simulink model "Woodward_v9_milestone"  (Simulink 7.8)
settings: Solver=ode5  StartTime=0.0  StopTime=inf  FixedStep=Ts  MaxStep=1e-3  RelTol=1e-3
PostLoadFcn:
  | Ts=50e-6;
InitFcn:
  | Ts=50e-6;
undefined symbols (not defined in the file): another_event_name, dfilt, DiscIntNeverNeededParam, fdesignblkfcn, gcbh, Gen_900kW_external_control, HIL_GenSet, Left, my_event_name, ph, type, V
libraries: simulink x66, powerlib x65, rtio_opalrt_common x21, powerlib_extras x20, dspsigops x10, simulink_extras x6, cables_lib x5, discretizing x4, rteventslib x4, dsparch4 x4, rtlab x3, ssn_lib x2
(part 1 of 5)
settings Model: ARTEMISmethode_block_infos=$$__separator__$$  Creator=CH24070  LastModifiedBy=ma25949  BufferReuse=off
settings SolverCC: ZeroCrossAlgorithm=Adaptive
settings DataIOCC: ExternalInput=getinputstruct(op_snapshot1)  InitialState=getstatestruct(op_snapshot1)  LimitDataPoints=off  MaxDataPoints=90060  SignalLoggingSaveFormat=Dataset  SaveOutput=off  SignalLogging=off  DSMLogging=off  SaveTime=off  OutputSaveName=result
settings OptimizationCC: BlockReduction=off  OptimizeBlockIOStorage=off  BufferReuse=off  ExpressionFolding=off  LocalBlockOutputs=off
settings DebuggingCC: MaxConsecutiveZCsMsg=warning  IgnoredZcDiagnostic=none  SolverPrmCheckMsg=none  MultiTaskRateTransMsg=warning  FrameProcessingCompatibilityMsg=error  ModelReferenceExtraNoncontSigs=warning
settings ModelReferenceCC: UpdateModelReferenceTargets=IfOutOfDate
settings SFSimCC: SFSimEcho=off
settings CodeAppCC: CustomSymbolStrType=$N$R$M_T
settings GRTTargetCC: TargetFunctionLibrary=C89/C90 (ANSI)
settings CustomProperty: DataType=string  Value=0

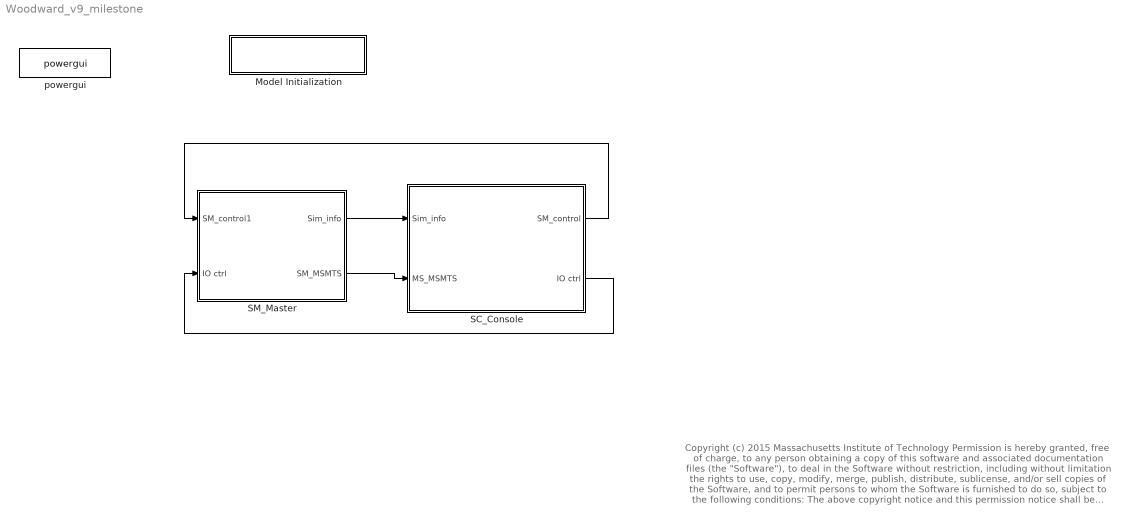
== system Woodward_v9_milestone ==
  note: Copyright (c) 2015 Massachusetts Institute of Technology
      | Permission is hereby granted, free of charge, to any person obtaining a copy of this software and associated documentation files (the "Software"), to deal in the Software without restriction, including without limitation the rights to use, copy, modify, merge, publish, distribute, sublicense, and/or sell copies of the Software, and to permit persons to whom the Software is furnished to do so, subject to the following conditions:
      |
      | The above copyright notice and this permission notice shall be included in all copies or substantial portions of the Software.
      |
      | THE SOFTWARE IS PROVIDED "AS IS", WITHOUT WARRANTY OF ANY KIND, EXPRESS OR IMPLIED, INCLUDING BUT NOT LIMITED TO THE WARRANTIES OF MERCHANTABILITY, FITNESS FOR A PARTICULAR PURPOSE AND NONINFRINGEMENT. IN NO EVENT SHALL THE AUTHORS OR COPYRIGHT HOLDERS BE LIABLE FOR ANY CLAIM,
      | DAMAGES OR OTHER LIABILITY, WHETHER IN AN ACTION OF CONTRACT, TORT OR OTHERWISE, ARISING FROM, OUT OF OR IN CONNECTION WITH THE SOFTWARE OR THE USE OR OTHER DEALINGS IN THE SOFTWARE.
  Model Initialization : Subsystem  AncestorBlock=artemis/Tools /Misc/Model Initialization  mask(Model Functions){InitFcnX=Ts=50e-6;, prel=off, posl=on, inif=on, strf=off}
      mask prompts: InitFcnX "Initialisation"; prel "Preload Function"; posl "PostLoad Function"; inif "InitFcn"; strf "StartFcn"
      mask init:
      | currentBlock = gcb;
      | root = bdroot(currentBlock);
      | 
      | if ~strcmp(get_param(root,'BlockDiagramType'),'library')
      |     if prel==1
      |         set_param(root, 'PreLoadFcn', InitFcnX);
      |     else
      |         set_param(root, 'PreLoadFcn', '');
      |     end
      |     if inif==1
      |         set_param(root, 'InitFcn', InitFcnX);
      |     else
      |         set_param(root, 'InitFcn', '');
      |     end
      |     if strf==1
      |         set_param(root, 'StartFcn', InitFcnX);
      |     else
      |         set_param(root, 'StartFcn', '');
      |     end
      |     if posl==1
      |         set_param(root, 'PostLoadFcn', InitFcnX);
      |     else
      |         set_param(root, 'PostLoadFcn', '');
      |     end
      | end
      | 
      | pos = get_param(currentBlock, 'Position');
      | width = pos(3) - pos(1); height = pos(4) - pos(2);
      | txt = [ upper(root) '\n' '- InitFcn. . . . . '  get_param(root, 'InitFcn') ];
      settings: CopyFcn=set_param(gcb,'LinkStatus','inactive')
      mask Display: text(5, height*0.5, txt, 'horizontalAlignment', 'left', 'verticalAlignment', 'middle') ;
  SC_Console : Subsystem
  SM_Master : Subsystem
  powergui : powerlib/powergui  Priority=2  SimulationMode=Discrete  SolverType=Tustin  SampleTime=Ts  frequency=60  SPID=off  DisableSnubberDevices=off  DisableRonSwitches=off  DisableVfSwitches=off  SwTol=0  Interpol=off  DisplayEquations=off  FunctionMessages=off  frequencyindice=0  Pbase=100e6  ErrMax=1e-4  Iterations=50  UnitsV=kV  UnitsW=MW  echomessages=off  HookPort=off  EnableUseOfTLC=off  x0status=blocks  RestoreLinks=warning  ResistiveCurrentMeasurement=off  Frange=logspace(0,3,50)  Ylog=off  Xlog=off  ShowGrid=off  save=off  variable=ZData  structure=0  ZoomFFT=on  StartTime=0.0  cycles=2  DisplayStyle=off  fundamental=60  FreqAxis=off  MaxFrequency=1000  frequencyindicesteady=1  RmsSteady=1  display=off  Ts=0  methode=off
  wires:
  SM_Master/1(Sim_info) -> SC_Console/1(Sim_info)
  SM_Master/2(SM_MSMTS) -> SC_Console/2(MS_MSMTS)
  SC_Console/1(SM_control) -> SM_Master/1(SM_control1)
  SC_Console/2(IO ctrl) -> SM_Master/2(IO ctrl)

== system Woodward_v9_milestone/Model Initialization ==

== system Woodward_v9_milestone/SC_Console ==
  note: Tcomputation
      | Ttotal
      | Idle
      | Overruns
  note: The 'Overruns' value should remain at 0.
      | The 'Ttotal' value should be equal to the
      | model Fixed-Step size.
  Sim_info : Inport
  MS_MSMTS : Inport  Port=2
  Bus Creator : BusCreator  Inputs=2
  Bus Selector : BusSelector  OutputSignals=Grid_PRM,Mains1_PRM,GEN_1MVA_PRM,Mains2_PRM,GEN_4MVA_PRM,Gen1_meas,Gen2_meas,Digital In,Load1,Load2,Load3
  Bus Selector{1..8} (8 alike) : BusSelector  OutputSignals=Grid_Status,sel_787.Grid_Vabc,sel_787.Iabc,sel_787.Grid_P,sel_787.Grid_Q
  Demux5 : Demux  Outputs=[1 8 4]
  Gen1_1MVA : Subsystem  AncestorBlock=HIL_GenSet/Gen_900kW_external_control
  Gen2_4MVA : Subsystem  AncestorBlock=HIL_GenSet/Gen_900kW_external_control
  OpComm : rtlab/OpComm  nbport=2  groupe_acq=1  subsys_rate=0  st=0  Synchronization=on  Interpolation=on  Threshold=1.0  Missed_Data=off  Sim_Time=off  Samples=off  dynSigOut=off  from_console=0  warning_done=off  writeOpCommFile=off  Offset=off
  Scope Gen1 : Scope  NumInputPorts=5
      settings: TimeRange=60  YMin=0~-600~-2000~-1000000~-1000000  YMax=1~600~2000~1000000~1000000
  Scope Gen2 : Scope  NumInputPorts=5
      settings: TimeRange=60  YMin=0~-20000~-20000~-1000000~-1000000  YMax=1~20000~20000~4000000~4000000  SaveName=ScopeData8
  Scope Grid : Scope  NumInputPorts=5
      settings: TimeRange=60  YMin=0~-20000~-20000~-1000000~-1000000  YMax=1~20000~20000~4000000~4000000  SaveName=ScopeData7
  Scope Load1 : Scope  NumInputPorts=5
      settings: TimeRange=60  YMin=0~-600~-2000~-1000000~-1000000  YMax=1~600~2000~1000000~1000000  SaveName=ScopeData6
  Scope Load2 : Scope  NumInputPorts=5
      settings: TimeRange=60  YMin=0~-600~-2000~-1000000~-1000000  YMax=1~600~2000~1000000~1000000  SaveName=ScopeData11
  Scope Load3 : Scope  NumInputPorts=5
      settings: TimeRange=60  YMin=0~-600~-2000~-1000000~-1000000  YMax=1~600~2000~1000000~1000000  SaveName=ScopeData10
  Scope Mains1 : Scope  NumInputPorts=5
      settings: TimeRange=60  YMin=0~-20000~-20000~-1000000~-1000000  YMax=1~20000~20000~4000000~4000000  SaveName=ScopeData5
  Scope Mains2 : Scope  NumInputPorts=5
      settings: TimeRange=60  YMin=0~-20000~-20000~-1000000~-1000000  YMax=1~20000~20000~4000000~4000000  SaveName=ScopeData9
  Status Codes : Display
      settings: Decimation=100
  TimingValues : Display
      settings: Decimation=100
  Woodward : Subsystem
  SM_control : Outport
  IO ctrl : Outport  Port=2
  wires:
  Sim_info/1 -> OpComm/1
  MS_MSMTS/1 -> OpComm/2
  Gen1_1MVA/1(S) -> Bus Creator/1  "Gen1_1MVA"
  Bus Creator/1 -> SM_control/1
  OpComm/2 -> Bus Selector/1
  Demux5/3 -> TimingValues/1
  OpComm/1 -> Demux5/1
  Demux5/1 -> Status Codes/1
  Woodward/1(Out1) -> IO ctrl/1
  Bus Selector1/1 -> Scope Grid/1  "<Grid_Status>"
  Bus Selector1/2 -> Scope Grid/2  "<Grid_Vabc>"
  Bus Selector1/3 -> Scope Grid/3  "<Iabc>"
  Bus Selector1/4 -> Scope Grid/4  "<Grid_P>"
  Bus Selector1/5 -> Scope Grid/5  "<Grid_Q>"
  Bus Selector2/1 -> Scope Mains1/1  "<Grid_Status>"
  Bus Selector2/2 -> Scope Mains1/2  "<Grid_Vabc>"
  Bus Selector2/3 -> Scope Mains1/3  "<Iabc>"
  Bus Selector2/4 -> Scope Mains1/4  "<Grid_P>"
  Bus Selector2/5 -> Scope Mains1/5  "<Grid_Q>"
  Bus Selector/1 -> Bus Selector1/1  "<Grid_PRM>"
  Bus Selector/2 -> Bus Selector2/1  "<Mains1_PRM>"
  Bus Selector3/1 -> Scope Load1/1  "<Grid_Status>"
  Bus Selector3/2 -> Scope Load1/2  "<Grid_Vabc>"
  Bus Selector3/3 -> Scope Load1/3  "<Iabc>"
  Bus Selector3/4 -> Scope Load1/4  "<Grid_P>"
  Bus Selector3/5 -> Scope Load1/5  "<Grid_Q>"
  Bus Selector/9 -> Bus Selector3/1  "<Load1>"
  Bus Selector4/1 -> Scope Gen1/1  "<Grid_Status>"
  Bus Selector4/2 -> Scope Gen1/2  "<Grid_Vabc>"
  Bus Selector4/3 -> Scope Gen1/3  "<Iabc>"
  Bus Selector4/4 -> Scope Gen1/4  "<Grid_P>"
  Bus Selector4/5 -> Scope Gen1/5  "<Grid_Q>"
  Bus Selector/3 -> Bus Selector4/1  "<GEN_1MVA_PRM>"
  Bus Selector5/1 -> Scope Gen2/1  "<Grid_Status>"
  Bus Selector5/2 -> Scope Gen2/2  "<Grid_Vabc>"
  Bus Selector5/3 -> Scope Gen2/3  "<Iabc>"
  Bus Selector5/4 -> Scope Gen2/4  "<Grid_P>"
  Bus Selector5/5 -> Scope Gen2/5  "<Grid_Q>"
  Bus Selector/5 -> Bus Selector5/1  "<GEN_4MVA_PRM>"
  Bus Selector/6 -> Woodward/1(Gen1_Primary)  "<Gen1_meas>"
  Bus Selector/8 -> Woodward/3(DIn_Ch00_31)  "<Digital In>"
  Bus Selector/7 -> Woodward/2(Gen2_Primary)  "<Gen2_meas>"
  Gen2_4MVA/1(S) -> Bus Creator/2  "Gen2_4MVA"
  Bus Selector6/1 -> Scope Mains2/1  "<Grid_Status>"
  Bus Selector6/2 -> Scope Mains2/2  "<Grid_Vabc>"
  Bus Selector6/3 -> Scope Mains2/3  "<Iabc>"
  Bus Selector6/4 -> Scope Mains2/4  "<Grid_P>"
  Bus Selector/4 -> Bus Selector6/1  "<Mains2_PRM>"
  Bus Selector6/5 -> Scope Mains2/5  "<Grid_Q>"
  Bus Selector7/1 -> Scope Load3/1  "<Grid_Status>"
  Bus Selector7/2 -> Scope Load3/2  "<Grid_Vabc>"
  Bus Selector7/3 -> Scope Load3/3  "<Iabc>"
  Bus Selector7/4 -> Scope Load3/4  "<Grid_P>"
  Bus Selector7/5 -> Scope Load3/5  "<Grid_Q>"
  Bus Selector8/1 -> Scope Load2/1  "<Grid_Status>"
  Bus Selector8/2 -> Scope Load2/2  "<Grid_Vabc>"
  Bus Selector8/3 -> Scope Load2/3  "<Iabc>"
  Bus Selector8/4 -> Scope Load2/4  "<Grid_P>"
  Bus Selector8/5 -> Scope Load2/5  "<Grid_Q>"
  Bus Selector/11 -> Bus Selector7/1  "<Load3>"
  Bus Selector/10 -> Bus Selector8/1  "<Load2>"

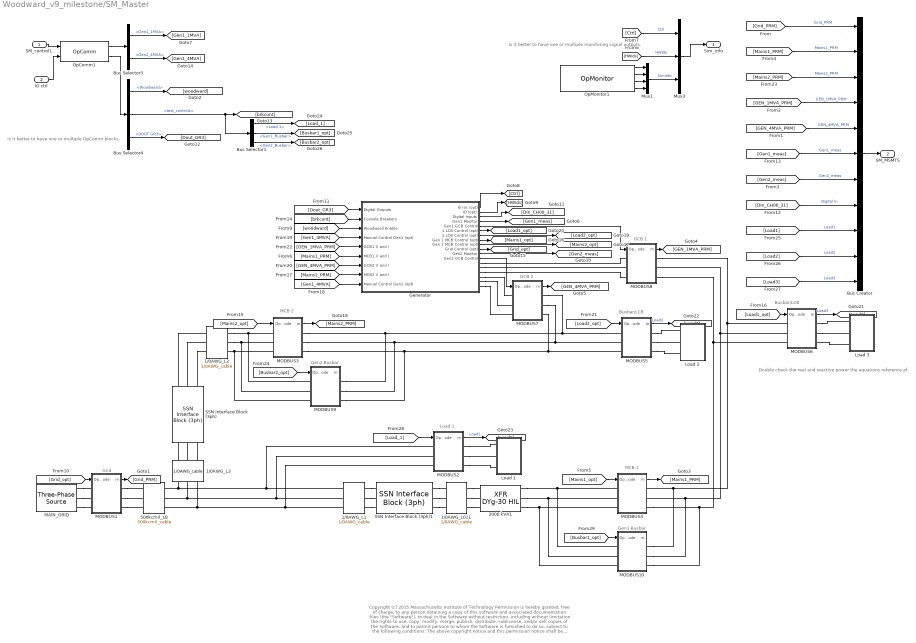
== system Woodward_v9_milestone/SM_Master ==
  note: Double check the real and reactive power
      | the equations reference pf.
  note: Is it better to have one
      | or multiple OpComm blocks.
  note: Is it better to have one or multiple
      | monitoring signal outputs.
  note: GCB 1
  note: Busbar/LCB
  note: MCB 1
  note: Grid
  note: MCB 2
  note: GCB 2
  note: Load 1
  note: Busbar/LCB
  note: Gen2 Busbar
  note: Gen1 Busbar
  note: Copyright (c) 2015 Massachusetts Institute of Technology
      | Permission is hereby granted, free of charge, to any person obtaining a copy of this software and associated documentation files (the "Software"), to deal in the Software without restriction, including without limitation the rights to use, copy, modify, merge, publish, distribute, sublicense, and/or sell copies of the Software, and to permit persons to whom the Software is furnished to do so, subject to the following conditions:
      |
      | The above copyright notice and this permission notice shall be included in all copies or substantial portions of the Software.
      |
      | THE SOFTWARE IS PROVIDED "AS IS", WITHOUT WARRANTY OF ANY KIND, EXPRESS OR IMPLIED, INCLUDING BUT NOT LIMITED TO THE WARRANTIES OF MERCHANTABILITY, FITNESS FOR A PARTICULAR PURPOSE AND NONINFRINGEMENT. IN NO EVENT SHALL THE AUTHORS OR COPYRIGHT HOLDERS BE LIABLE FOR ANY CLAIM,
      | DAMAGES OR OTHER LIABILITY, WHETHER IN AN ACTION OF CONTRACT, TORT OR OTHERWISE, ARISING FROM, OUT OF OR IN CONNECTION WITH THE SOFTWARE OR THE USE OR OTHER DEALINGS IN THE SOFTWARE.
  SM_control1 : Inport
  IO ctrl : Inport  Port=2
  1/0AWG_L011 : cables_lib/1//0AWG_cable  length=1000  par_sets=1
  1/0AWG_L1 : cables_lib/1//0AWG_cable  length=1  par_sets=1
  1/0AWG_L2 : cables_lib/1//0AWG_cable  length=1  par_sets=1
  1/0AWG_L3 : cables_lib/1//0AWG_cable  length=1  par_sets=1
  2000 kVA1 : transformer_lib/XFR DYg-30 HIL  Rating=2000  Vp=13800  Vs=480  Z=5.75  XR=5.7
  500kcmil_L8 : cables_lib/500kcmil_cable  length=1  par_sets=1
  Bus Creator : BusCreator  Inputs=11
  Bus Selector1 : BusSelector  OutputSignals=Load 1,Gen1_Busbar,Gen2_Busbar
  Bus Selector3 : BusSelector  OutputSignals=Gen1_1MVA,Gen2_4MVA
  Bus Selector4 : BusSelector  OutputSignals=Woodward,test_controls,DOUT GR3
  Generator : Subsystem
  Load 1 : Subsystem  mask{v=13800, kVA=1000, pf=0.90}
      mask prompts: v "VRMSLL"
  Load 2 : Subsystem  mask{v=13800, kVA=2000, pf=0.90}
      mask prompts: v "VRMSLL"
  Load 3 : Subsystem  mask{v=480, kVA=500, pf=0.90}
      mask prompts: v "VRMSLL"
  MAIN_GRID : powerlib/Electrical Sources/Three-Phase Source  Voltage=13800  PhaseAngle=0  Frequency=60  InternalConnection=Yg  SpecifyImpedance=on  Resistance=0.8929  Inductance=16.58e-3  ShortCircuitLevel=375e6  BaseVoltage=13800  XRratio=7.9  BusType=swing  Pref=0  Qref=0  Qmin=-inf  Qmax=inf
  MODBUS1 : Subsystem  mask(Protection and Metering){IOC=15E3, TOC=1800, Ts=Ts, VRMSLL=13800, I_nom=200}
      mask prompts: IOC "IOC setting [A]"; TOC "TOC setting [A]"; Ts "Sampling Time [Sec]"; VRMSLL "Nominal Voltage [VRMSLL]"; I_nom "Continous Current [A]"
      mask help:
      | This block simulates the behavior of selected relay functions as well as metering equipment.
      | The block is intended to communicate with a microgrid controller providing it measurements, and switching controls.
      mask Help:
      | This block simulates the behavior of selected relay functions as well as metering equipment (60 Hz - only).
      | The block is intended to communicate with a microgrid controller providing it measurements, and switching controls.
      | 
      | The input parameters are:
      | 0) Ts:  Sampling time [Seconds]
      | 1) State: 0 for relay logic mode, 1 to close the controlled breaker/switch,
      | and 2 to open the controlled breaker/switch
      | 2) TOC: Time-inverse overcurrent setting [Amperes]
      | 3) IOC: Instantaneous overcurrent setting [Amperes]
      | 
      | Metered parameters are:
      | 0) Status (0-closed, 1-open)
      | 1) Instantaneous voltage (abc)
      | 2) Instantaneous current (abc)
  MODBUS10 : Subsystem  mask(Protection and Metering){IOC=15E3, TOC=1800, Ts=Ts, VRMSLL=480, I_nom=2000}
      mask prompts: IOC "IOC setting [A]"; TOC "TOC setting [A]"; Ts "Sampling Time [Sec]"; VRMSLL "Nominal Voltage [VRMSLL]"; I_nom "Continous Current [A]"
      mask help:
      | This block simulates the behavior of selected relay functions as well as metering equipment.
      | The block is intended to communicate with a microgrid controller providing it measurements, and switching controls.
      mask Help:
      | This block simulates the behavior of selected relay functions as well as metering equipment (60 Hz - only).
      | The block is intended to communicate with a microgrid controller providing it measurements, and switching controls.
      | 
      | The input parameters are:
      | 0) Ts:  Sampling time [Seconds]
      | 1) State: 0 for relay logic mode, 1 to close the controlled breaker/switch,
      | and 2 to open the controlled breaker/switch
      | 2) TOC: Time-inverse overcurrent setting [Amperes]
      | 3) IOC: Instantaneous overcurrent setting [Amperes]
      | 
      | Metered parameters are:
      | 0) Status (0-closed, 1-open)
      | 1) Instantaneous voltage (abc)
      | 2) Instantaneous current (abc)
  MODBUS2 : Subsystem  mask(Protection and Metering){IOC=15E3, TOC=1800, Ts=Ts, VRMSLL=13800, I_nom=200}
      mask prompts: IOC "IOC setting [A]"; TOC "TOC setting [A]"; Ts "Sampling Time [Sec]"; VRMSLL "Nominal Voltage [VRMSLL]"; I_nom "Continous Current [A]"
      mask help:
      | This block simulates the behavior of selected relay functions as well as metering equipment.
      | The block is intended to communicate with a microgrid controller providing it measurements, and switching controls.
      mask Help:
      | This block simulates the behavior of selected relay functions as well as metering equipment (60 Hz - only).
      | The block is intended to communicate with a microgrid controller providing it measurements, and switching controls.
      | 
      | 
      | The input parameters are:
      | 0) Ts:  Sampling time [Seconds]
      | 1) State: 0 for relay logic mode, 1 to close the controlled breaker/switch,
      | and 2 to open the controlled breaker/switch
      | 2) TOC: Time-inverse overcurrent setting [Amperes]
      | 3) IOC: Instantaneous overcurrent setting [Amperes]
      | 
      | Metered parameters are:
      | 0) Status (0-closed, 1-open)
      | 1) Instantaneous voltage (abc)
      | 2) Instantaneous current (abc)
  MODBUS3 : Subsystem  mask(Protection and Metering){IOC=15E3, TOC=1800, Ts=Ts, VRMSLL=13800, I_nom=200}
      mask prompts: IOC "IOC setting [A]"; TOC "TOC setting [A]"; Ts "Sampling Time [Sec]"; VRMSLL "Nominal Voltage [VRMSLL]"; I_nom "Continous Current [A]"
      mask help:
      | This block simulates the behavior of selected relay functions as well as metering equipment.
      | The block is intended to communicate with a microgrid controller providing it measurements, and switching controls.
      mask Help:
      | This block simulates the behavior of selected relay functions as well as metering equipment (60 Hz - only).
      | The block is intended to communicate with a microgrid controller providing it measurements, and switching controls.
      | 
      | The input parameters are:
      | 0) Ts:  Sampling time [Seconds]
      | 1) State: 0 for relay logic mode, 1 to close the controlled breaker/switch,
      | and 2 to open the controlled breaker/switch
      | 2) TOC: Time-inverse overcurrent setting [Amperes]
      | 3) IOC: Instantaneous overcurrent setting [Amperes]
      | 
      | Metered parameters are:
      | 0) Status (0-closed, 1-open)
      | 1) Instantaneous voltage (abc)
      | 2) Instantaneous current (abc)
  MODBUS4 : Subsystem  mask(Protection and Metering){IOC=15E3, TOC=1800, Ts=Ts, VRMSLL=480, I_nom=2000}
      mask prompts: IOC "IOC setting [A]"; TOC "TOC setting [A]"; Ts "Sampling Time [Sec]"; VRMSLL "Nominal Voltage [VRMSLL]"; I_nom "Continous Current [A]"
      mask help:
      | This block simulates the behavior of selected relay functions as well as metering equipment.
      | The block is intended to communicate with a microgrid controller providing it measurements, and switching controls.
      mask Help:
      | This block simulates the behavior of selected relay functions as well as metering equipment (60 Hz - only).
      | The block is intended to communicate with a microgrid controller providing it measurements, and switching controls.
      | 
      | The input parameters are:
      | 0) Ts:  Sampling time [Seconds]
      | 1) State: 0 for relay logic mode, 1 to close the controlled breaker/switch,
      | and 2 to open the controlled breaker/switch
      | 2) TOC: Time-inverse overcurrent setting [Amperes]
      | 3) IOC: Instantaneous overcurrent setting [Amperes]
      | 
      | Metered parameters are:
      | 0) Status (0-closed, 1-open)
      | 1) Instantaneous voltage (abc)
      | 2) Instantaneous current (abc)
  MODBUS5 : Subsystem  mask(Protection and Metering){IOC=15E3, TOC=1800, Ts=Ts, VRMSLL=13800, I_nom=200}
      mask prompts: IOC "IOC setting [A]"; TOC "TOC setting [A]"; Ts "Sampling Time [Sec]"; VRMSLL "Nominal Voltage [VRMSLL]"; I_nom "Continous Current [A]"
      mask help:
      | This block simulates the behavior of selected relay functions as well as metering equipment.
      | The block is intended to communicate with a microgrid controller providing it measurements, and switching controls.
      mask Help:
      | This block simulates the behavior of selected relay functions as well as metering equipment (60 Hz - only).
      | The block is intended to communicate with a microgrid controller providing it measurements, and switching controls.
      | 
      | The input parameters are:
      | 0) Ts:  Sampling time [Seconds]
      | 1) State: 0 for relay logic mode, 1 to close the controlled breaker/switch,
      | and 2 to open the controlled breaker/switch
      | 2) TOC: Time-inverse overcurrent setting [Amperes]
      | 3) IOC: Instantaneous overcurrent setting [Amperes]
      | 
      | Metered parameters are:
      | 0) Status (0-closed, 1-open)
      | 1) Instantaneous voltage (abc)
      | 2) Instantaneous current (abc)
  MODBUS6 : Subsystem  mask(Protection and Metering){IOC=15E3, TOC=1800, Ts=Ts, VRMSLL=13800, I_nom=200}
      mask prompts: IOC "IOC setting [A]"; TOC "TOC setting [A]"; Ts "Sampling Time [Sec]"; VRMSLL "Nominal Voltage [VRMSLL]"; I_nom "Continous Current [A]"
      mask help:
      | This block simulates the behavior of selected relay functions as well as metering equipment.
      | The block is intended to communicate with a microgrid controller providing it measurements, and switching controls.
      mask Help:
      | This block simulates the behavior of selected relay functions as well as metering equipment (60 Hz - only).
      | The block is intended to communicate with a microgrid controller providing it measurements, and switching controls.
      | 
      | The input parameters are:
      | 0) Ts:  Sampling time [Seconds]
      | 1) State: 0 for relay logic mode, 1 to close the controlled breaker/switch,
      | and 2 to open the controlled breaker/switch
      | 2) TOC: Time-inverse overcurrent setting [Amperes]
      | 3) IOC: Instantaneous overcurrent setting [Amperes]
      | 
      | Metered parameters are:
      | 0) Status (0-closed, 1-open)
      | 1) Instantaneous voltage (abc)
      | 2) Instantaneous current (abc)
  MODBUS7 : Subsystem  mask(Protection and Metering){IOC=15E3, TOC=1800, Ts=Ts, VRMSLL=13800, I_nom=200}
      mask prompts: IOC "IOC setting [A]"; TOC "TOC setting [A]"; Ts "Sampling Time [Sec]"; VRMSLL "Nominal Voltage [VRMSLL]"; I_nom "Continous Current [A]"
      mask help:
      | This block simulates the behavior of selected relay functions as well as metering equipment.
      | The block is intended to communicate with a microgrid controller providing it measurements, and switching controls.
      mask Help:
      | This block simulates the behavior of selected relay functions as well as metering equipment (60 Hz - only).
      | The block is intended to communicate with a microgrid controller providing it measurements, and switching controls.
      | 
      | The input parameters are:
      | 0) Ts:  Sampling time [Seconds]
      | 1) State: 0 for relay logic mode, 1 to close the controlled breaker/switch,
      | and 2 to open the controlled breaker/switch
      | 2) TOC: Time-inverse overcurrent setting [Amperes]
      | 3) IOC: Instantaneous overcurrent setting [Amperes]
      | 
      | Metered parameters are:
      | 0) Status (0-closed, 1-open)
      | 1) Instantaneous voltage (abc)
      | 2) Instantaneous current (abc)
  MODBUS8 : Subsystem  mask(Protection and Metering){IOC=15E3, TOC=1800, Ts=Ts, VRMSLL=480, I_nom=2000}
      mask prompts: IOC "IOC setting [A]"; TOC "TOC setting [A]"; Ts "Sampling Time [Sec]"; VRMSLL "Nominal Voltage [VRMSLL]"; I_nom "Continous Current [A]"
      mask help:
      | This block simulates the behavior of selected relay functions as well as metering equipment.
      | The block is intended to communicate with a microgrid controller providing it measurements, and switching controls.
      mask Help:
      | This block simulates the behavior of selected relay functions as well as metering equipment (60 Hz - only).
      | The block is intended to communicate with a microgrid controller providing it measurements, and switching controls.
      | 
      | The input parameters are:
      | 0) Ts:  Sampling time [Seconds]
      | 1) State: 0 for relay logic mode, 1 to close the controlled breaker/switch,
      | and 2 to open the controlled breaker/switch
      | 2) TOC: Time-inverse overcurrent setting [Amperes]
      | 3) IOC: Instantaneous overcurrent setting [Amperes]
      | 
      | Metered parameters are:
      | 0) Status (0-closed, 1-open)
      | 1) Instantaneous voltage (abc)
      | 2) Instantaneous current (abc)
  MODBUS9 : Subsystem  mask(Protection and Metering){IOC=15E3, TOC=1800, Ts=Ts, VRMSLL=13800, I_nom=200}
      mask prompts: IOC "IOC setting [A]"; TOC "TOC setting [A]"; Ts "Sampling Time [Sec]"; VRMSLL "Nominal Voltage [VRMSLL]"; I_nom "Continous Current [A]"
      mask help:
      | This block simulates the behavior of selected relay functions as well as metering equipment.
      | The block is intended to communicate with a microgrid controller providing it measurements, and switching controls.
      mask Help:
      | This block simulates the behavior of selected relay functions as well as metering equipment (60 Hz - only).
      | The block is intended to communicate with a microgrid controller providing it measurements, and switching controls.
      | 
      | 
      | The input parameters are:
      | 0) Ts:  Sampling time [Seconds]
      | 1) State: 0 for relay logic mode, 1 to close the controlled breaker/switch,
      | and 2 to open the controlled breaker/switch
      | 2) TOC: Time-inverse overcurrent setting [Amperes]
      | 3) IOC: Instantaneous overcurrent setting [Amperes]
      | 
      | Metered parameters are:
      | 0) Status (0-closed, 1-open)
      | 1) Instantaneous voltage (abc)
      | 2) Instantaneous current (abc)
  Mux1 : Mux
  Mux3 : Mux  Inputs=[1 8 4]
  OpComm1 : rtlab/OpComm  nbport=2  groupe_acq=1  subsys_rate=0  st=0  Synchronization=on  Interpolation=on  Threshold=1.0  Missed_Data=off  Sim_Time=off  Samples=off  dynSigOut=off  from_console=1  warning_done=off  writeOpCommFile=off  Offset=off
  OpMonitor1 : rtlab/Monitoring/OpMonitor  compute_time=on  real_step=on  idle_time=on  nb_overruns=on  user_time=off  user_name=my_event_name,another_event_name
  SSN Interface Block (3ph) : ssn_lib/SSN Interface Block (3ph)  nb_phase=3  nb_port=2  p1_type=V-type(Left)  p2_type=V-type (Right)  p3_type=V-type(Left)  p4_type=V-type(Left)  p5_type=V-type(Left)  p6_type=V-type(Left)  p7_type=V-type(Left)  p8_type=V-type(Left)  p9_type=V-type(Left)  p10_type=V-type(Left)  p11_type=V-type(Left)  p12_type=V-type(Left)  p13_type=V-type(Left)  p14_type=V-type(Left)  p15_type=V-type(Left)  p16_type=V-type(Left)  I_port_shunt_resistance=1e9
  SSN Interface Block (3ph)1 : ssn_lib/SSN Interface Block (3ph)  nb_phase=3  nb_port=2  p1_type=V-type(Left)  p2_type=V-type (Right)  p3_type=V-type(Left)  p4_type=V-type(Left)  p5_type=V-type(Left)  p6_type=V-type(Left)  p7_type=V-type(Left)  p8_type=V-type(Left)  p9_type=V-type(Left)  p10_type=V-type(Left)  p11_type=V-type(Left)  p12_type=V-type(Left)  p13_type=V-type(Left)  p14_type=V-type(Left)  p15_type=V-type(Left)  p16_type=V-type(Left)  I_port_shunt_resistance=1e9
  Sim_info : Outport
  SM_MSMTS : Outport  Port=2
  wires:
  [Grid_PRM] -> Bus Creator/1  "Grid_PRM"
  [GEN_1MVA_PRM] -> Bus Creator/4  "GEN_1MVA_PRM"
  [Mains1_PRM] -> Bus Creator/2  "Mains1_PRM"
  Bus Creator/1 -> SM_MSMTS/1
  SM_control1/1 -> OpComm1/1
  OpComm1/1 -> Bus Selector3/1
  Bus Selector3/1 -> [Gen1_1MVA]  "<Gen1_1MVA>"
  OpComm1/2 -> Bus Selector4/1
  Bus Selector4/1 -> [woodward]  "<Woodward>"
  IO ctrl/1 -> OpComm1/2
  Bus Selector4/3 -> [Dout_GR3]  "<DOUT GR3>"
  OpMonitor1/1 -> Mux1/1
  OpMonitor1/2 -> Mux1/2
  OpMonitor1/3 -> Mux1/3
  OpMonitor1/4 -> Mux1/4
  Mux1/1 -> Mux3/3  "SimInfo"
  [Ctrl] -> Mux3/1  "Ctrl"
  [HWIds] -> Mux3/2  "HWIds"
  Mux3/1 -> Sim_info/1
  Bus Selector4/2 -> [brkcont], Bus Selector1/1  "<test_controls>"
  MODBUS1/1(m) -> [Grid_PRM]
  MODBUS8/1(m) -> [GEN_1MVA_PRM]
  [Dout_GR3] -> Generator/1(Digital Outputs)
  [brkcont] -> Generator/2(Console Breakers)
  Generator/4(Gen1 Monitor) -> [Gen1_meas]
  Generator/1(Error (opt)) -> [Ctrl]
  Generator/2(ID (opt)) -> [HWIds]
  Generator/3(Digital Inputs) -> [DIn_CH00_31]
  [Gen1_4MVA] -> Generator/4(Manual Control Gen1 (opt))
  [woodward] -> Generator/3(Woodward Enable)
  Generator/5(Gen1 GCB Control) -> MODBUS8/1(Op_Mode)
  Generator/12(Gen2 GCB Control) -> MODBUS7/1(Op_Mode)
  [GEN_4MVA_PRM] -> Bus Creator/5  "GEN_4MVA_PRM"
  Generator/11(Gen2 Monitor) -> [Gen2_meas]
  [Gen1_meas] -> Bus Creator/6  "Gen1_meas"
  [Gen2_meas] -> Bus Creator/7  "Gen2_meas"
  [DIn_CH00_31] -> Bus Creator/8  "Digital In"
  Bus Selector3/2 -> [Gen1_4MVA]  "<Gen2_4MVA>"
  [Gen1_4MVA] -> Generator/9(Manual Control Gen2 (opt))
  Generator/10(Grid Control (opt)) -> [Grid_opt]
  [Grid_opt] -> MODBUS1/1(Op_Mode)
  Generator/8(Gen 1 MCB Control (opt)) -> [Mains1_opt]
  Generator/9(Gen 2 MCB Control (opt)) -> [Mains2_opt]
  [Mains2_opt] -> MODBUS3/1(Op_Mode)
  MODBUS3/1(m) -> [Mains2_PRM]
  [Mains2_PRM] -> Generator/8(MCB2 V and I)
  [Mains1_PRM] -> Generator/6(MCB1 V and I)
  Generator/7(2 LCB Control (opt)) -> [Load2_opt]
  Generator/6(1 LCB Control (opt)) -> [Load1_opt]
  MODBUS7/1(m) -> [GEN_4MVA_PRM]
  [GEN_4MVA_PRM] -> Generator/7(GCB2 V and I)
  [GEN_1MVA_PRM] -> Generator/5(GCB1 V and I)
  [Mains2_PRM] -> Bus Creator/3  "Mains2_PRM"
  MODBUS4/1(m) -> [Mains1_PRM]
  [Mains1_opt] -> MODBUS4/1(Op_Mode)
  [Load2_opt] -> MODBUS5/1(Op_Mode)
  [Load1_opt] -> MODBUS6/1(Op_Mode)
  MODBUS2/1(m) -> [Load1]  "Load1"
  MODBUS5/1(m) -> [Load2]  "Load2"
  MODBUS6/1(m) -> [Load3]  "Load3"
  [Load1] -> Bus Creator/9  "Load1"
  [Load2] -> Bus Creator/10  "Load2"
  [Load3] -> Bus Creator/11  "Load3"
  Bus Selector1/1 -> [Load_1]  "<Load 1>"
  Bus Selector1/2 -> [Busbar1_opt]  "<Gen1_Busbar>"
  Bus Selector1/3 -> [Busbar2_opt]  "<Gen2_Busbar>"
  [Busbar2_opt] -> MODBUS9/1(Op_Mode)
  [Load_1] -> MODBUS2/1(Op_Mode)
  [Busbar1_opt] -> MODBUS10/1(Op_Mode)
  connections:
  1/0AWG_L011/RConn1 -- 2000 kVA1/LConn1
  1/0AWG_L011/RConn2 -- 2000 kVA1/LConn2
  1/0AWG_L011/RConn3 -- 2000 kVA1/LConn3
  1/0AWG_L1/LConn1 -- MODBUS2/LConn1 -- 500kcmil_L8/RConn1 -- 1/0AWG_L3/LConn1
  1/0AWG_L1/LConn2 -- MODBUS2/LConn2 -- 500kcmil_L8/RConn2 -- 1/0AWG_L3/LConn2
  1/0AWG_L1/LConn3 -- MODBUS2/LConn3 -- 500kcmil_L8/RConn3 -- 1/0AWG_L3/LConn3
  MODBUS4/RConn3 -- MODBUS6/LConn3 -- MODBUS8/RConn3 -- MODBUS10/RConn3
  MODBUS1/RConn3 -- 500kcmil_L8/LConn3
  MODBUS1/RConn2 -- 500kcmil_L8/LConn2
  MODBUS1/RConn1 -- 500kcmil_L8/LConn1
  MAIN_GRID/RConn3 -- MODBUS1/LConn3
  MAIN_GRID/RConn2 -- MODBUS1/LConn2
  MAIN_GRID/RConn1 -- MODBUS1/LConn1
  Generator/RConn3 -- MODBUS8/LConn3
  Generator/RConn2 -- MODBUS8/LConn2
  Generator/RConn1 -- MODBUS8/LConn1
  Generator/RConn6 -- MODBUS7/LConn3
  Generator/RConn5 -- MODBUS7/LConn2
  Generator/RConn4 -- MODBUS7/LConn1
  MODBUS2/RConn3 -- Load 1/LConn3
  MODBUS2/RConn2 -- Load 1/LConn2
  MODBUS2/RConn1 -- Load 1/LConn1
  MODBUS6/LConn2 -- MODBUS8/RConn2 -- MODBUS4/RConn2 -- MODBUS10/RConn2
  MODBUS6/LConn1 -- MODBUS8/RConn1 -- MODBUS4/RConn1 -- MODBUS10/RConn1
  MODBUS3/RConn3 -- MODBUS5/LConn3 -- MODBUS7/RConn3 -- MODBUS9/RConn3
  MODBUS3/RConn2 -- MODBUS5/LConn2 -- MODBUS7/RConn2 -- MODBUS9/RConn2
  MODBUS3/RConn1 -- MODBUS5/LConn1 -- MODBUS7/RConn1 -- MODBUS9/RConn1
  2000 kVA1/RConn3 -- MODBUS4/LConn3 -- MODBUS10/LConn3
  2000 kVA1/RConn2 -- MODBUS4/LConn2 -- MODBUS10/LConn2
  2000 kVA1/RConn1 -- MODBUS4/LConn1 -- MODBUS10/LConn1
  MODBUS5/RConn3 -- Load 2/LConn3
  MODBUS5/RConn2 -- Load 2/LConn2
  MODBUS5/RConn1 -- Load 2/LConn1
  MODBUS6/RConn3 -- Load 3/LConn3
  MODBUS6/RConn2 -- Load 3/LConn2
  MODBUS6/RConn1 -- Load 3/LConn1
  SSN Interface Block (3ph)1/RConn1 -- 1/0AWG_L011/LConn1
  SSN Interface Block (3ph)1/RConn2 -- 1/0AWG_L011/LConn2
  SSN Interface Block (3ph)1/RConn3 -- 1/0AWG_L011/LConn3
  1/0AWG_L1/RConn3 -- SSN Interface Block (3ph)1/LConn3
  1/0AWG_L1/RConn2 -- SSN Interface Block (3ph)1/LConn2
  1/0AWG_L1/RConn1 -- SSN Interface Block (3ph)1/LConn1
  MODBUS9/LConn3 -- MODBUS3/LConn3 -- 1/0AWG_L2/RConn3
  MODBUS9/LConn2 -- MODBUS3/LConn2 -- 1/0AWG_L2/RConn2
  MODBUS9/LConn1 -- MODBUS3/LConn1 -- 1/0AWG_L2/RConn1
  SSN Interface Block (3ph)/RConn3 -- 1/0AWG_L2/LConn3
  SSN Interface Block (3ph)/RConn2 -- 1/0AWG_L2/LConn2
  SSN Interface Block (3ph)/RConn1 -- 1/0AWG_L2/LConn1
  1/0AWG_L3/RConn3 -- SSN Interface Block (3ph)/LConn3
  1/0AWG_L3/RConn2 -- SSN Interface Block (3ph)/LConn2
  1/0AWG_L3/RConn1 -- SSN Interface Block (3ph)/LConn1

== system Woodward_v9_milestone/SC_Console/Gen1_1MVA ==
  1 - PQ 2 - PV 3 - VF : Constant  Value=3
  Bus Creator : BusCreator  Inputs=6
  DONOTCHANGE : Constant
  Enable = 1 Disable = 0 : Constant  Value=0
  F : simulink/Math Operations/Slider Gain  low=0.97  gain=1  high=1.03
  P : simulink/Math Operations/Slider Gain  low=0  gain=0.8  high=1.1
  Q : simulink/Math Operations/Slider Gain  low=0.01  gain=0.2  high=0.4
  V : simulink/Math Operations/Slider Gain  low=0.9  gain=1  high=1.1
  S : Outport
  wires:
  DONOTCHANGE/1 -> P/1, Q/1, V/1, F/1
  Bus Creator/1 -> S/1
  P/1 -> Bus Creator/1  "P"
  Q/1 -> Bus Creator/2  "Q"
  V/1 -> Bus Creator/3  "V"
  F/1 -> Bus Creator/4  "F"
  1 - PQ 2 - PV 3 - VF/1 -> Bus Creator/5  "Mode"
  Enable = 1 Disable = 0/1 -> Bus Creator/6  "Enable"

== system Woodward_v9_milestone/SC_Console/Gen2_4MVA ==
  1 - PQ 2 - PV 3 - VF : Constant  Value=3
  Bus Creator : BusCreator  Inputs=6
  DONOTCHANGE : Constant
  Enable = 1 Disable = 0 : Constant  Value=0
  F : simulink/Math Operations/Slider Gain  low=0.97  gain=1  high=1.03
  P : simulink/Math Operations/Slider Gain  low=0  gain=0.8  high=1.1
  Q : simulink/Math Operations/Slider Gain  low=0.01  gain=0.2  high=0.4
  V : simulink/Math Operations/Slider Gain  low=0.9  gain=1  high=1.1
  S : Outport
  wires:
  DONOTCHANGE/1 -> P/1, Q/1, V/1, F/1
  Bus Creator/1 -> S/1
  P/1 -> Bus Creator/1  "P"
  Q/1 -> Bus Creator/2  "Q"
  V/1 -> Bus Creator/3  "V"
  F/1 -> Bus Creator/4  "F"
  1 - PQ 2 - PV 3 - VF/1 -> Bus Creator/5  "Mode"
  Enable = 1 Disable = 0/1 -> Bus Creator/6  "Enable"

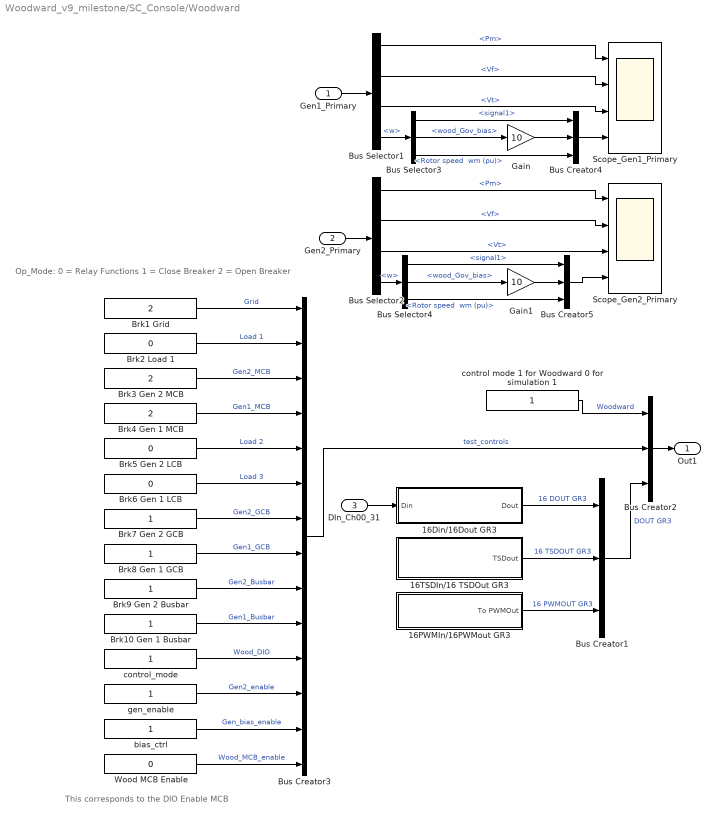
== system Woodward_v9_milestone/SC_Console/Woodward ==
  note: Op_Mode:
      | 0 = Relay Functions
      | 1 = Close Breaker
      | 2 = Open Breaker
  note: This corresponds to
      | the DIO Enable MCB
  Gen1_Primary : Inport
  Gen2_Primary : Inport  Port=2
  DIn_Ch00_31 : Inport  Port=3
  16Din/16Dout GR3 : Subsystem
  16PWMIn/16PWMout GR3 : Subsystem
  16TSDIn/16 TSDOut GR3 : Subsystem
  Brk1 Grid : Constant  Value=2
  Brk10 Gen 1 Busbar : Constant
  Brk2 Load 1 : Constant  Value=0
  Brk3 Gen 2 MCB : Constant  Value=2
  Brk4 Gen 1 MCB : Constant  Value=2
  Brk5 Gen 2 LCB : Constant  Value=0
  Brk6 Gen 1 LCB : Constant  Value=0
  Brk7 Gen 2 GCB : Constant
  Brk8 Gen 1 GCB : Constant
  Brk9 Gen 2 Busbar : Constant
  Bus Creator{1..2,4..5} (4 alike) : BusCreator  Inputs=3
  Bus Creator3 : BusCreator  Inputs=14
  Bus Selector1 : BusSelector  OutputSignals=Pm,Vf,Vt,w
  Bus Selector2 : BusSelector  OutputSignals=Pm,Vf,Vt,w
  Bus Selector3 : BusSelector  OutputSignals="signal1,w.wood_Gov_bias,w.Rotor speed  wm (pu)"
  Bus Selector4 : BusSelector  OutputSignals="signal1,w.wood_Gov_bias,w.Rotor speed  wm (pu)"
  Gain : Gain  Gain=10
  Gain1 : Gain  Gain=10
  Scope_Gen1_Primary : Scope  NumInputPorts=4
      settings: TimeRange=60  YMin=0~-5~-1~-1  YMax=1.1~5~2~2  SaveName=ScopeData4
  Scope_Gen2_Primary : Scope  NumInputPorts=4
      settings: TimeRange=60  YMin=0~-5~-1~-1  YMax=1.1~5~2~2  SaveName=ScopeData3
  Wood MCB Enable : Constant  Value=0
  bias_ctrl : Constant
  control mode 1 for Woodward 0 for simulation 1 : Constant
  control_mode : Constant
  gen_enable : Constant
  Out1 : Outport
  wires:
  control mode 1 for Woodward 0 for simulation 1/1 -> Bus Creator2/1  "Woodward"
  16Din/16Dout GR3/1(Dout) -> Bus Creator1/1  "16 DOUT GR3"
  16TSDIn/16 TSDOut GR3/1(TSDout) -> Bus Creator1/2  "16 TSDOUT GR3"
  16PWMIn/16PWMout GR3/1(To PWMOut) -> Bus Creator1/3  "16 PWMOUT GR3"
  Bus Creator1/1 -> Bus Creator2/3  "DOUT GR3"
  Bus Creator3/1 -> Bus Creator2/2  "test_controls"
  Brk1 Grid/1 -> Bus Creator3/1  "Grid"
  Brk2 Load 1/1 -> Bus Creator3/2  "Load 1"
  Brk3 Gen 2 MCB/1 -> Bus Creator3/3  "Gen2_MCB"
  Brk4 Gen 1 MCB/1 -> Bus Creator3/4  "Gen1_MCB"
  control_mode/1 -> Bus Creator3/11  "Wood_DIO"
  gen_enable/1 -> Bus Creator3/12  "Gen2_enable"
  bias_ctrl/1 -> Bus Creator3/13  "Gen_bias_enable"
  Bus Creator2/1 -> Out1/1
  DIn_Ch00_31/1 -> 16Din/16Dout GR3/1(Din)
  Bus Selector1/1 -> Scope_Gen1_Primary/1  "<Pm>"
  Bus Selector1/2 -> Scope_Gen1_Primary/2  "<Vf>"
  Bus Selector1/3 -> Scope_Gen1_Primary/3  "<Vt>"
  Gen1_Primary/1 -> Bus Selector1/1
  Wood MCB Enable/1 -> Bus Creator3/14  "Wood_MCB_enable"
  Gen2_Primary/1 -> Bus Selector2/1
  Bus Selector2/1 -> Scope_Gen2_Primary/1  "<Pm>"
  Bus Selector2/2 -> Scope_Gen2_Primary/2  "<Vf>"
  Bus Selector2/3 -> Scope_Gen2_Primary/3  "<Vt>"
  Bus Selector1/4 -> Bus Selector3/1  "<w>"
  Bus Selector3/1 -> Bus Creator4/1  "<signal1>"
  Bus Selector3/2 -> Gain/1  "<wood_Gov_bias>"
  Bus Selector3/3 -> Bus Creator4/3  "<Rotor speed  wm (pu)>"
  Bus Creator4/1 -> Scope_Gen1_Primary/4
  Bus Selector4/1 -> Bus Creator5/1  "<signal1>"
  Bus Selector4/2 -> Gain1/1  "<wood_Gov_bias>"
  Bus Selector4/3 -> Bus Creator5/3  "<Rotor speed  wm (pu)>"
  Bus Selector2/4 -> Bus Selector4/1  "<w>"
  Bus Creator5/1 -> Scope_Gen2_Primary/4
  Brk5 Gen 2 LCB/1 -> Bus Creator3/5  "Load 2"
  Brk6 Gen 1 LCB/1 -> Bus Creator3/6  "Load 3"
  Brk7 Gen 2 GCB/1 -> Bus Creator3/7  "Gen2_GCB"
  Brk8 Gen 1 GCB/1 -> Bus Creator3/8  "Gen1_GCB"
  Gain1/1 -> Bus Creator5/2
  Gain/1 -> Bus Creator4/2
  Brk9 Gen 2 Busbar/1 -> Bus Creator3/9  "Gen2_Busbar"
  Brk10 Gen 1 Busbar/1 -> Bus Creator3/10  "Gen1_Busbar"

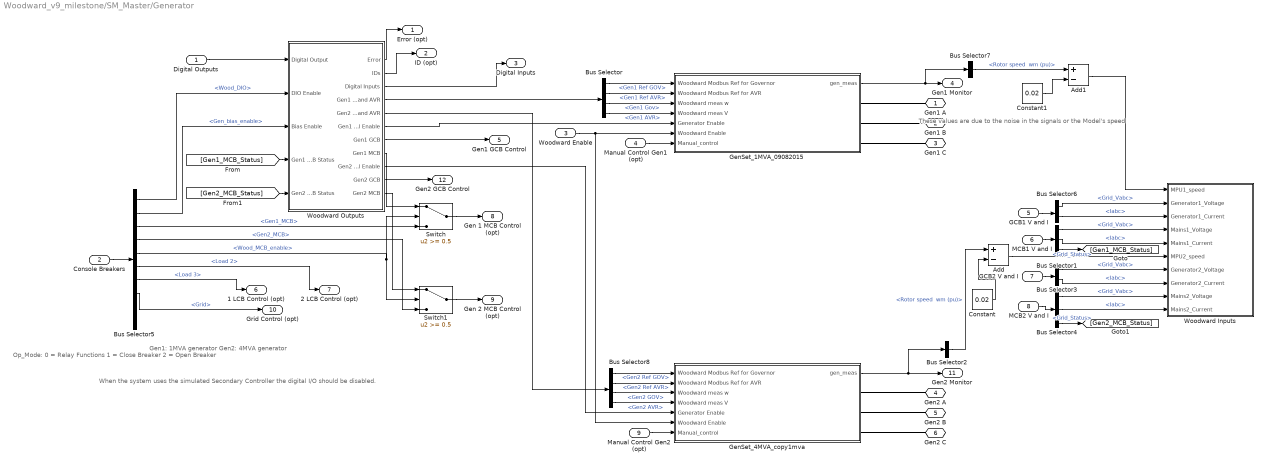
== system Woodward_v9_milestone/SM_Master/Generator ==
  note: Op_Mode:
      | 0 = Relay Functions
      | 1 = Close Breaker
      | 2 = Open Breaker
  note: These values are due to
      | the noise in the signals
      | or the Model's speed
  note: Gen1: 1MVA generator
      | Gen2: 4MVA generator
  note: When the system uses the simulated
      | Secondary Controller the digital I/O
      | should be disabled.
  Digital Outputs : Inport
  Console Breakers : Inport  Port=2
  Woodward Enable : Inport  Port=3
  Manual Control Gen1 (opt) : Inport  Port=4
  GCB1 V and I : Inport  Port=5
  MCB1 V and I : Inport  Port=6
  GCB2 V and I : Inport  Port=7
  MCB2 V and I : Inport  Port=8
  Manual Control Gen2 (opt) : Inport  Port=9
  Add : Sum  Inputs=+-
  Add1 : Sum  Inputs=+-
  Bus Selector : BusSelector  OutputSignals=Gen1 Ref GOV,Gen1 Ref AVR,Gen1 Gov,Gen1 AVR
  Bus Selector1 : BusSelector  OutputSignals=sel_787.Grid_Vabc,sel_787.Iabc,Grid_Status
  Bus Selector2 : BusSelector  OutputSignals="w.w.Rotor speed  wm (pu)"
  Bus Selector3 : BusSelector  OutputSignals=sel_787.Grid_Vabc,sel_787.Iabc
  Bus Selector4 : BusSelector  OutputSignals=sel_787.Grid_Vabc,sel_787.Iabc,Grid_Status
  Bus Selector5 : BusSelector  OutputSignals=Wood_DIO,Gen_bias_enable,Gen1_MCB,Gen2_MCB,Wood_MCB_enable,Load 2,Load 3,Grid,Gen2_enable,Load 1
  Bus Selector6 : BusSelector  OutputSignals=sel_787.Grid_Vabc,sel_787.Iabc
  Bus Selector7 : BusSelector  OutputSignals="w.w.Rotor speed  wm (pu)"
  Bus Selector8 : BusSelector  OutputSignals=Gen2 Ref GOV,Gen2 Ref AVR,Gen2 GOV,Gen2 AVR
  Constant : Constant  Value=0.02
  Constant1 : Constant  Value=0.02
  GenSet_1MVA_09082015 : Subsystem  mask(Gen-Set with simulated control modes){control_mode=1}
      mask prompts: control_mode "Control Mode [0 => Sim. 1 => Wood.]"
      mask help:
      | This Gen-Set block allows the user to indicate the control mode of the generator. The available control modes are: (1) PQ, (2) PV, and (3) VF.
      | The input values to the block will be applied according to the selected control mode.
      | For example, if PQ mode is selected, the controller will only work based on P_ref and Q_ref ignoring values of other inputs to the block.
  GenSet_4MVA_copy1mva : Subsystem  mask(Gen-Set with simulated control modes){control_mode=1}
      mask prompts: control_mode "Control Mode [0 => Sim. 1 => Wood.]"
      mask help:
      | This Gen-Set block allows the user to indicate the control mode of the generator. The available control modes are: (1) PQ, (2) PV, and (3) VF.
      | The input values to the block will be applied according to the selected control mode.
      | For example, if PQ mode is selected, the controller will only work based on P_ref and Q_ref ignoring values of other inputs to the block.
  Switch : Switch  Threshold=0.5
  Switch1 : Switch  Threshold=0.5
  Woodward Inputs : Subsystem
  Woodward Outputs : Subsystem
  Gen1 A : PMIOPort  Port=1  Side=Right
  Gen1 B : PMIOPort  Port=2  Side=Right
  Gen1 C : PMIOPort  Port=3  Side=Right
  Gen2 A : PMIOPort  Port=4  Side=Right
  Gen2 B : PMIOPort  Port=5  Side=Right
  Gen2 C : PMIOPort  Port=6  Side=Right
  Error (opt) : Outport
  ID (opt) : Outport  Port=2
  Digital Inputs : Outport  Port=3
  Gen1 Monitor : Outport  Port=4
  Gen1 GCB Control : Outport  Port=5
  1 LCB Control (opt) : Outport  Port=6
  2 LCB Control (opt) : Outport  Port=7
  Gen 1 MCB Control (opt) : Outport  Port=8
  Gen 2 MCB Control (opt) : Outport  Port=9
  Grid Control (opt) : Outport  Port=10
  Gen2 Monitor : Outport  Port=11
  Gen2 GCB Control : Outport  Port=12
  wires:
  GenSet_1MVA_09082015/1(gen_meas) -> Bus Selector7/1, Gen1 Monitor/1
  Bus Selector6/1 -> Woodward Inputs/2(Generator1_Voltage)  "<Grid_Vabc>"
  Bus Selector6/2 -> Woodward Inputs/3(Generator1_Current)  "<Iabc>"
  Bus Selector5/1 -> Woodward Outputs/2(DIO Enable)  "<Wood_DIO>"
  Manual Control Gen1 (opt)/1 -> GenSet_1MVA_09082015/7(Manual_control)
  Bus Selector5/2 -> Woodward Outputs/3(Bias Enable)  "<Gen_bias_enable>"
  Bus Selector7/1 -> Add1/1  "<Rotor speed  wm (pu)>"
  Woodward Outputs/1(Error) -> Error (opt)/1
  Woodward Outputs/2(IDs) -> ID (opt)/1
  Woodward Outputs/3(Digital Inputs) -> Digital Inputs/1
  Woodward Enable/1 -> GenSet_1MVA_09082015/6(Woodward Enable), GenSet_4MVA_copy1mva/6(Woodward Enable)
  Woodward Outputs/6(Gen1 Fuel Enable) -> GenSet_1MVA_09082015/5(Generator Enable)
  Bus Selector5/5 -> Switch/2, Switch1/2  "<Wood_MCB_enable>"
  Woodward Outputs/8(Gen1 MCB) -> Switch/1
  Digital Outputs/1 -> Woodward Outputs/1(Digital Output)
  GCB1 V and I/1 -> Bus Selector6/1
  Woodward Outputs/7(Gen1 GCB) -> Gen1 GCB Control/1
  Console Breakers/1 -> Bus Selector5/1
  Bus Selector5/7 -> 1 LCB Control (opt)/1  "<Load 3>"
  Switch/1 -> Gen 1 MCB Control (opt)/1
  MCB1 V and I/1 -> Bus Selector1/1
  Bus Selector1/1 -> Woodward Inputs/4(Mains1_Voltage)  "<Grid_Vabc>"
  Bus Selector1/2 -> Woodward Inputs/5(Mains1_Current)  "<Iabc>"
  GCB2 V and I/1 -> Bus Selector3/1
  MCB2 V and I/1 -> Bus Selector4/1
  GenSet_4MVA_copy1mva/1(gen_meas) -> Gen2 Monitor/1, Bus Selector2/1
  Bus Selector2/1 -> Add/1  "<Rotor speed  wm (pu)>"
  Bus Selector3/1 -> Woodward Inputs/7(Generator2_Voltage)  "<Grid_Vabc>"
  Bus Selector3/2 -> Woodward Inputs/8(Generator2_Current)  "<Iabc>"
  Bus Selector4/1 -> Woodward Inputs/9(Mains2_Voltage)  "<Grid_Vabc>"
  Bus Selector4/2 -> Woodward Inputs/10(Mains2_Current)  "<Iabc>"
  Woodward Outputs/4(Gen1 Gov and AVR) -> Bus Selector/1
  Bus Selector/1 -> GenSet_1MVA_09082015/1(Woodward Modbus Ref for Governor)  "<Gen1 Ref GOV>"
  Bus Selector/2 -> GenSet_1MVA_09082015/2(Woodward Modbus Ref for AVR)  "<Gen1 Ref AVR>"
  Bus Selector/3 -> GenSet_1MVA_09082015/3(Woodward meas w)  "<Gen1 Gov>"
  Bus Selector/4 -> GenSet_1MVA_09082015/4(Woodward meas V)  "<Gen1 AVR>"
  Woodward Outputs/5(Gen2 Gov and AVR) -> Bus Selector8/1
  Bus Selector8/1 -> GenSet_4MVA_copy1mva/1(Woodward Modbus Ref for Governor)  "<Gen2 Ref GOV>"
  Bus Selector8/2 -> GenSet_4MVA_copy1mva/2(Woodward Modbus Ref for AVR)  "<Gen2 Ref AVR>"
  Bus Selector8/3 -> GenSet_4MVA_copy1mva/3(Woodward meas w)  "<Gen2 GOV>"
  Bus Selector8/4 -> GenSet_4MVA_copy1mva/4(Woodward meas V)  "<Gen2 AVR>"
  Manual Control Gen2 (opt)/1 -> GenSet_4MVA_copy1mva/7(Manual_control)
  Woodward Outputs/9(Gen2 Fuel Enable) -> GenSet_4MVA_copy1mva/5(Generator Enable)
  Woodward Outputs/10(Gen2 GCB) -> Gen2 GCB Control/1
  Add/1 -> Woodward Inputs/6(MPU2_speed)
  Constant/1 -> Add/2
  Bus Selector1/3 -> [Gen1_MCB_Status]  "<Grid_Status>"
  Bus Selector4/3 -> [Gen2_MCB_Status]  "<Grid_Status>"
  [Gen1_MCB_Status] -> Woodward Outputs/4(Gen1 MCB Status)
  [Gen2_MCB_Status] -> Woodward Outputs/5(Gen2 MCB Status)
  Switch1/1 -> Gen 2 MCB Control (opt)/1
  Woodward Outputs/11(Gen2 MCB) -> Switch1/1
  Bus Selector5/6 -> 2 LCB Control (opt)/1  "<Load 2>"
  Bus Selector5/4 -> Switch1/3  "<Gen2_MCB>"
  Bus Selector5/3 -> Switch/3  "<Gen1_MCB>"
  Bus Selector5/8 -> Grid Control (opt)/1  "<Grid>"
  Constant1/1 -> Add1/2
  Add1/1 -> Woodward Inputs/1(MPU1_speed)
  connections:
  Gen1 A/RConn1 -- GenSet_1MVA_09082015/RConn1
  Gen1 B/RConn1 -- GenSet_1MVA_09082015/RConn2
  Gen1 C/RConn1 -- GenSet_1MVA_09082015/RConn3
  GenSet_4MVA_copy1mva/RConn1 -- Gen2 A/RConn1
  GenSet_4MVA_copy1mva/RConn2 -- Gen2 B/RConn1
  GenSet_4MVA_copy1mva/RConn3 -- Gen2 C/RConn1

== system Woodward_v9_milestone/SM_Master/Load 1 ==
  Constant Load : powerlib/Elements/Three-Phase Parallel RLC Load  LConnTagsString=A|B|C  Configuration=Y (grounded)  NominalVoltage=v  NominalFrequency=60  ActivePower=kVA*1E3*pf  InductivePower=kVA*1E3*sqrt(1-pf^2)  CapacitivePower=0  Measurements=None  LoadType=constant Z
  A : PMIOPort  Port=1  Side=Left
  B : PMIOPort  Port=2  Side=Left
  C : PMIOPort  Port=3  Side=Left
  connections:
  Constant Load/LConn1 -- A/RConn1
  B/RConn1 -- Constant Load/LConn2
  C/RConn1 -- Constant Load/LConn3

== system Woodward_v9_milestone/SM_Master/Load 2 ==
  Constant Load : powerlib/Elements/Three-Phase Parallel RLC Load  LConnTagsString=A|B|C  Configuration=Y (grounded)  NominalVoltage=v  NominalFrequency=60  ActivePower=kVA*1E3*pf  InductivePower=kVA*1E3*sqrt(1-pf^2)  CapacitivePower=0  Measurements=None  LoadType=constant Z
  A : PMIOPort  Port=1  Side=Left
  B : PMIOPort  Port=2  Side=Left
  C : PMIOPort  Port=3  Side=Left
  connections:
  Constant Load/LConn1 -- A/RConn1
  B/RConn1 -- Constant Load/LConn2
  C/RConn1 -- Constant Load/LConn3

== system Woodward_v9_milestone/SM_Master/Load 3 ==
  Constant Load : powerlib/Elements/Three-Phase Parallel RLC Load  LConnTagsString=A|B|C  Configuration=Y (grounded)  NominalVoltage=v  NominalFrequency=60  ActivePower=kVA*1E3*pf  InductivePower=kVA*1E3*sqrt(1-pf^2)  CapacitivePower=0  Measurements=None  LoadType=constant Z
  A : PMIOPort  Port=1  Side=Left
  B : PMIOPort  Port=2  Side=Left
  C : PMIOPort  Port=3  Side=Left
  connections:
  Constant Load/LConn1 -- A/RConn1
  B/RConn1 -- Constant Load/LConn2
  C/RConn1 -- Constant Load/LConn3
